simulink model "SensibleStorageExampleSim"  (R2020b)
settings: Solver=ode4  StartTime=0.0  StopTime=500  FixedStep=1e-2  RelTol=1e-3  EnableMultiTasking=on
undefined symbols (not defined in the file): sigbuilder_block
settings Model: Creator=chiavazzo  LastModifiedBy=chiavazzo
settings DataIOCC: ReturnWorkspaceOutputs=off
settings OptimizationCC: LifeSpan=inf
settings DebuggingCC: SFUnexpectedBacktrackingDiag=warning  SFNoUnconditionalDefaultTransitionDiag=warning  ArithmeticOperatorsInVariantConditions=warning
settings SFSimCC: SimUseLocalCustomCode=off  CustomCodeUndefinedFunction=UseInterfaceOnly
settings RTWCC: RTWUseLocalCustomCode=off
settings CodeAppCC: StateflowObjectComments=on
settings GRTTargetCC: TargetLangStandard=C89/C90 (ANSI)
settings ConfigComp: CovMetricSettings=dw  CovSaveCumulativeToWorkspaceVar=on  CovSaveSingleToWorkspaceVar=on  CovExternalEMLEnable=off

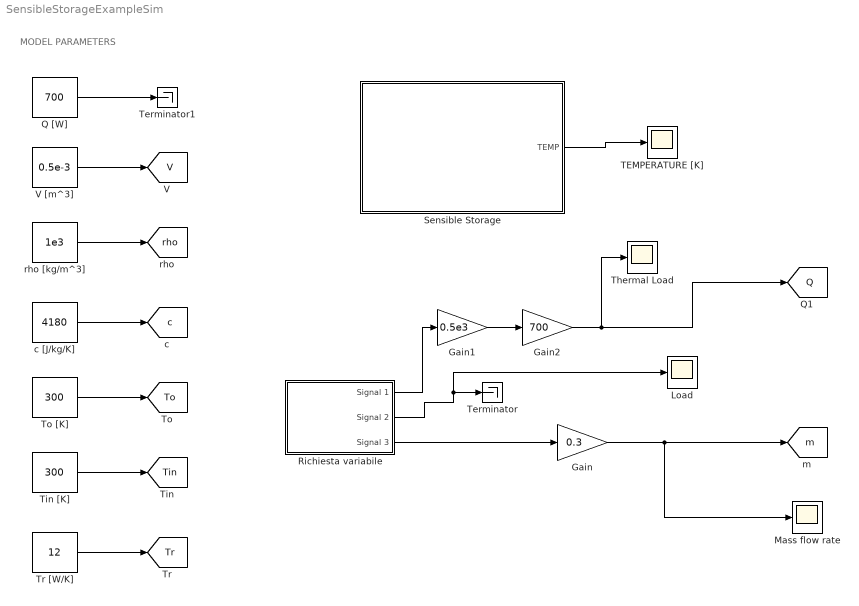
== system SensibleStorageExampleSim ==
  note: MODEL PARAMETERS
  Gain : Gain  Gain=0.3
  Gain1 : Gain  Gain=0.5e3
  Gain2 : Gain  Gain=700
  Load : Scope
  Mass flow rate : Scope
  Q [W] : Constant  Value=700
  Richiesta variabile : Subsystem  Tag=STV Subsys  LoadFcn=sigbuilder_block('load');  StartFcn=sigbuilder_block('start');  StopFcn=sigbuilder_block('stop');  ClipboardFcn=sigbuilder_block('clipboard');  mask(Sigbuilder block){tuvar=[0:10]}
      mask help: Simulink:masks:SigbuilderBlock_MD
      mask init:
      | if ~strcmp(get_param(bdroot(gcbh),'SimulationStatus'),'stopped') tuvar = sigbuilder_block('maskInit'); end
      settings: CopyFcn=sigbuilder_block('copy');  DeleteFcn=sigbuilder_block('delete');  ModelCloseFcn=sigbuilder_block('modelClose');  PreSaveFcn=sigbuilder_block('preSave');  PauseFcn=sigbuilder_block('pause');  ContinueFcn=sigbuilder_block('continue');  NameChangeFcn=sigbuilder_block('namechange');  OpenFcn=sigbuilder_block('open',[127.5 52 736 384 ]);  CloseFcn=sigbuilder_block('close');
      mask Display: plot(0, 0, 100, 100,[2, 2, 32, 32, 2], [68, 8, 8, 68, 68],[32, 2], [38, 38], [32, 19, 2],[53, 60, 44], [32, 17, 17, 2],[16, 16, 31, 31]);txt = getActiveGroup(gcbh);text(2, 100, txt,'verticalAlignment', 'top');
  Sensible Storage : Subsystem
  TEMPERATURE [K] : Scope
  Terminator : Terminator
  Terminator1 : Terminator
  Thermal Load : Scope
  Tin [K] : Constant  Value=300
  To [K] : Constant  Value=300
  Tr [W/K] : Constant  Value=12
  V [m^3] : Constant  Value=0.5e-3
  c [J/kg/K] : Constant  Value=4180
  rho [kg/m^3] : Constant  Value=1e3
  tag scope: Q=global, Tin=global, To=global, Tr=global, V=global, c=global, m=global, rho=global
  wires:
  V [m^3]/1 -> [V]
  rho [kg/m^3]/1 -> [rho]
  c [J/kg/K]/1 -> [c]
  To [K]/1 -> [To]
  Tin [K]/1 -> [Tin]
  Tr [W/K]/1 -> [Tr]
  Richiesta variabile/3(Signal 3) -> Gain/1
  Richiesta variabile/2(Signal 2) -> Load/1, Terminator/1
  Richiesta variabile/1(Signal 1) -> Gain1/1
  Sensible Storage/1(TEMP) -> TEMPERATURE [K]/1
  Gain/1 -> Mass flow rate/1, [m]
  Gain1/1 -> Gain2/1
  Gain2/1 -> Thermal Load/1, [Q]
  Q [W]/1 -> Terminator1/1

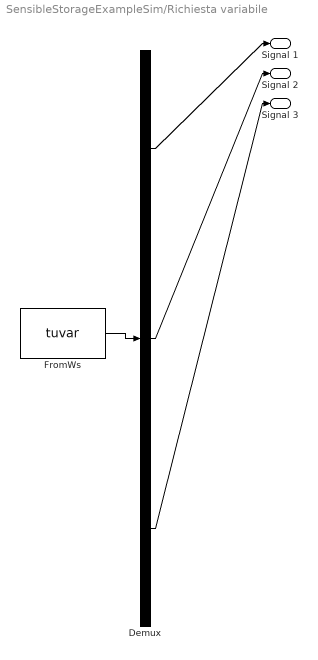
== system SensibleStorageExampleSim/Richiesta variabile ==
  Demux : Demux  Tag=STV Demux  Outputs=3
      settings: DisplayOption=none
  FromWs : FromWorkspace  Tag=STV FromWs  VariableName=tuvar
      SigBuilderData=|
      | common.afterFinalStr = 'Extrapolate'
      | common.sampleTime = 0
      | dataSet.timeRange = [0 500]
      | dataSet.name = 'Group 1'
      | sbobj.Groups.Name = 'Group 1'
      | sbobj.Groups.Signals(1).Name = 'Signal 1'
      | sbobj.Groups.Signals(1).XData = [0 10 10 20 20 30 30 40 40 50 50 60 60 70 70 80 80 90 90 100 100 110 110 120 120 130 130 140 140 150 150 160 160 170 170 180 180 190 190 200 200 210 210 220 220 230 230 240 240 250 250 260 260 270 270 280 280 290 290 300 300 310 310 320 320 330 330 340 340 350 350 360 360 370 370 380 380 390 390 400 400 410 410 420 420 430 430 440 440 450 450 460 460 470 470 480 480 490 490 500]
      | sbobj.Groups.Signals(1).YData = [0.002 0.002 0 0 0.002 0.002 0 0 0.002 0.002 0 0 0.002 0.002 0 0 0.002 0.002 0 0 0.002 0.002 0 0 0.002 0.002 0 0 0.002 0.002 0 0 0.002 0.002 0 0 0.002 0.002 0 0 0.002 0.002 0 0 0.002 0.002 0 0 0.002 0.002 0 0 0.002 0.002 0 0 0.002 0.002 0 0 0.002 0.002 0 0 0.002 0.002 0 0 0.002 0.002 0 0 0.002 0.002 0 0 0.002 0.002 0 0 0.002 0.002 0 0 0.002 0.002 0 0 0.002 0.002 0 0 0.002 0.002 0 0 0.002 0.002 0 0]
      | sbobj.Groups.Signals(2).Name = 'Signal 2'
      | sbobj.Groups.Signals(2).XData = [0 500]
      | sbobj.Groups.Signals(2).YData = [0 0]
      | sbobj.Groups.Signals(3).Name = 'Signal 3'
      | sbobj.Groups.Signals(3).XData = [0 50 50 100 100 150 150 200 200 250 250 300 300 350 350 400 400 450 450 500]
      | sbobj.Groups.Signals(3).YData = [0 0.08 0 0.08 0 0.08 0 0.08 0 0.08 0 0.08 0 0.08 0 0.08 0 0.08 0 0.08]
      | sbobj.Groups.TimeRange = [0 500]
  Signal 1 : Outport  Tag=STV Outport
  Signal 2 : Outport  Tag=STV Outport  Port=2
  Signal 3 : Outport  Tag=STV Outport  Port=3
  wires:
  FromWs/1 -> Demux/1
  Demux/1 -> Signal 1/1
  Demux/2 -> Signal 2/1
  Demux/3 -> Signal 3/1

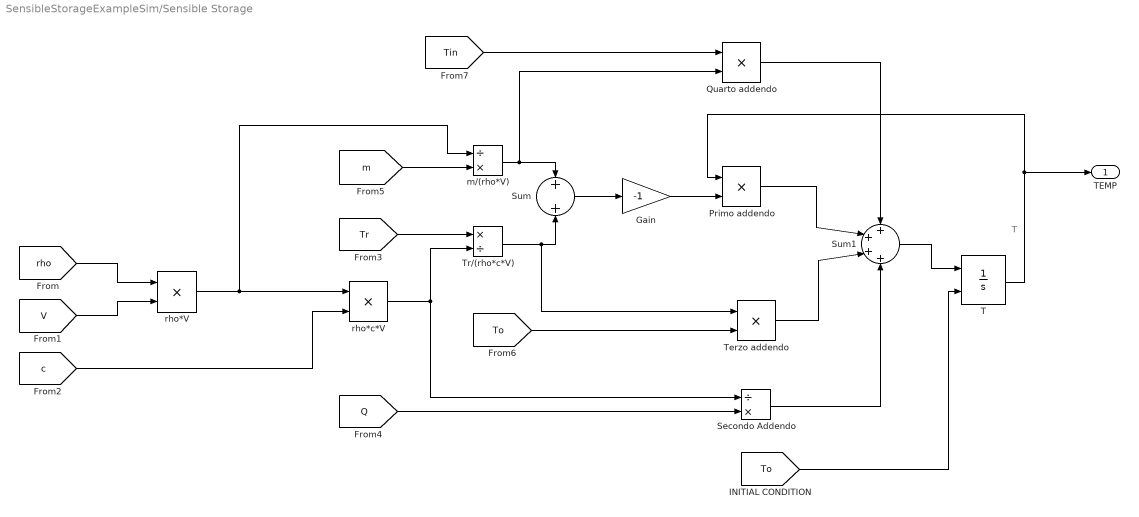
== system SensibleStorageExampleSim/Sensible Storage ==
  note: T
  Gain : Gain  Gain=-1
  Primo addendo : Product
  Quarto addendo : Product
  Secondo Addendo : Product  Inputs=/*
  Sum : Sum
  Sum1 : Sum  Inputs=4
  T : Integrator  InitialConditionSource=external
  Terzo addendo : Product
  Tr/(rho*c*V) : Product  Inputs=*/
  m/(rho*V) : Product  Inputs=/*
  rho*V : Product
  rho*c*V : Product
  TEMP : Outport
  wires:
  rho*V/1 -> m/(rho*V)/1, rho*c*V/1
  Secondo Addendo/1 -> Sum1/4
  [Q] -> Secondo Addendo/2
  [c] -> rho*c*V/2
  Tr/(rho*c*V)/1 -> Terzo addendo/1, Sum/2
  rho*c*V/1 -> Secondo Addendo/1, Tr/(rho*c*V)/2
  [Tr] -> Tr/(rho*c*V)/1
  [To] -> Terzo addendo/2
  Quarto addendo/1 -> Sum1/1
  [Tin] -> Quarto addendo/1
  [V] -> rho*V/2
  Sum/1 -> Gain/1
  Primo addendo/1 -> Sum1/2
  Gain/1 -> Primo addendo/2
  Terzo addendo/1 -> Sum1/3
  [rho] -> rho*V/1
  Sum1/1 -> T/1
  [To] -> T/2
  T/1 -> TEMP/1, Primo addendo/1
  m/(rho*V)/1 -> Sum/1, Quarto addendo/2
  [m] -> m/(rho*V)/2
